simulink model "interpolazione"  (R2018a)
settings: Solver=VariableStepAuto  StartTime=0.0  StopTime=5  RelTol=1e-3
libraries: dspvision x4, phasedwavlib x1
settings Model: Creator=116983  LastModifiedBy=stefa

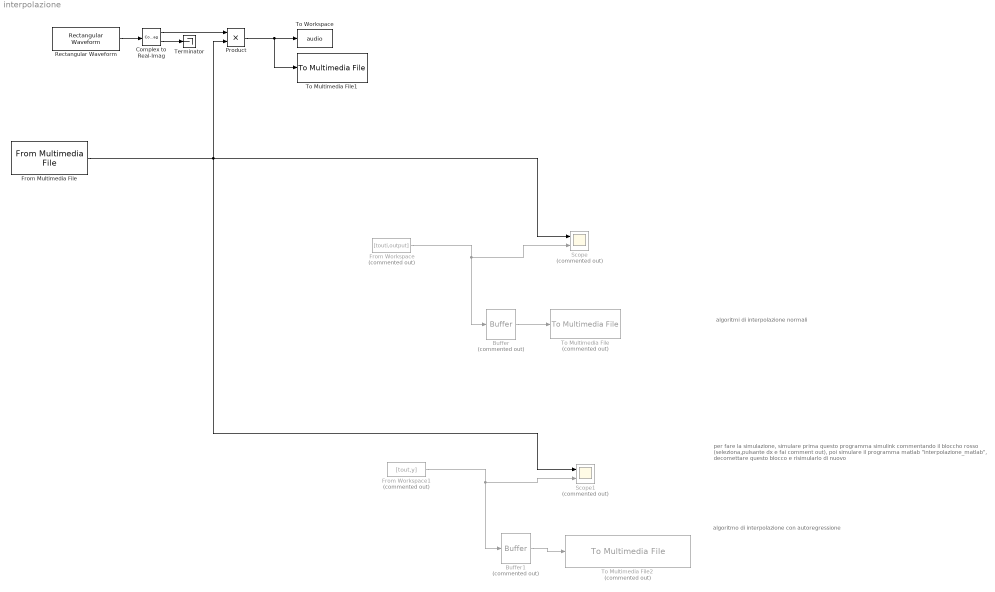
== system interpolazione ==
  note: algoritmo di interpolazione con autoregressione
  note: algoritmi di interpolazione normali
  note: per fare la simulazione, simulare prima questo programma simulink commentando il bloccho rosso (seleziona,pulsante dx e fai comment out), poi simulare il programma matlab "interpolazione_matlab", decomettare questo blocco e risimularlo di nuovo
  Buffer : Buffer  Commented=on  N=1024  OutputFrames=off
  Buffer1 : Buffer  Commented=on  N=1024  OutputFrames=off
  Complex to Real-Imag : ComplexToRealImag
  From Workspace : FromWorkspace  Commented=on  VariableName=[touti,output]  OutDataTypeStr=double  SampleTime=1/22050  Interpolate=off  OutputAfterFinalValue=Setting to zero
  From Workspace1 : FromWorkspace  Commented=on  VariableName=[tout,y]  OutDataTypeStr=double  SampleTime=1/22050  Interpolate=off  OutputAfterFinalValue=Setting to zero
  From Multimedia File : dspvision/From Multimedia File  inputFilename=speech_dft.mp3  loop=on  numPlays=inf  outputStreams=Audio only  videoDataType=single  audioDataType=double  inheritSampleTime=on  userDefinedSampleTime=1/8000  noAudioOutput=off  isIntensityVideo=off  fourcc=RGB  colorVideoFormat=Separate color signals  outputEOF=off  dataOrg=Column-major  audioFrameSize=1  computeAudioFrameSize=off  outSamplingMode=Sample based
      settings: SourceProductBaseCode=VP
  Product : Product  OutDataTypeStr=double  InputSameDT=on
  Rectangular Waveform : phasedwavlib/Rectangular Waveform  SampleRate=22050  DurationSpecification=Pulse width  PulseWidth=0.95  DutyCycle=0.5  PRF=1  PRFSelectionInputPort=off  OutputFormat=Samples  NumSamples=1  NumPulses=1  SimulateUsing=Interpreted execution
      settings: SourceProductName=Phased Array System Toolbox  SourceProductBaseCode=AR
  Scope : Scope  Commented=on  NumInputPorts=2
  Scope1 : Scope  Commented=on  NumInputPorts=2
  Terminator : Terminator
  To Multimedia File : dspvision/To Multimedia File  Commented=on  outputFilename=C:\Users\116983\Desktop\cubic.wav  streamSelection=Audio only  videoCompressor=None (uncompressed)  audioCompressor=None (uncompressed)  imagePorts=Separate color signals  fileType=WAV  audioDatatype=16-bit integer  fourcc=RGB  videoQuality=75  mj2000CompFactor=10
      settings: SourceProductName=Computer Vision System Toolbox  SourceProductBaseCode=VP
  To Multimedia File1 : dspvision/To Multimedia File  outputFilename=C:\Users\116983\Desktop\output2.wav  streamSelection=Audio only  videoCompressor=None (uncompressed)  audioCompressor=None (uncompressed)  imagePorts=Separate color signals  fileType=WAV  audioDatatype=16-bit integer  fourcc=RGB  videoQuality=75  mj2000CompFactor=10
      settings: SourceProductName=Computer Vision System Toolbox  SourceProductBaseCode=VP
  To Multimedia File2 : dspvision/To Multimedia File  Commented=on  outputFilename=C:\Users\116983\Desktop\interpolateAR.wav  streamSelection=Audio only  videoCompressor=None (uncompressed)  audioCompressor=None (uncompressed)  imagePorts=Separate color signals  fileType=WAV  audioDatatype=16-bit integer  fourcc=RGB  videoQuality=75  mj2000CompFactor=10
      settings: SourceProductName=Computer Vision System Toolbox  SourceProductBaseCode=VP
  To Workspace : ToWorkspace  VariableName=audio  SampleTime=-1
      settings: Save2DSignal=2-D array (concatenate along first dimension)
  wires:
  From Multimedia File/1 -> Scope1/1, Scope/1, Product/2
  Rectangular Waveform/1 -> Complex to Real-Imag/1
  Complex to Real-Imag/1 -> Product/1
  From Workspace/1 -> Scope/2, Buffer/1
  Complex to Real-Imag/2 -> Terminator/1
  Buffer/1 -> To Multimedia File/1
  Product/1 -> To Multimedia File1/1, To Workspace/1
  Buffer1/1 -> To Multimedia File2/1
  From Workspace1/1 -> Scope1/2, Buffer1/1
